simulink model "switch_sample"  (R2021a)
settings: Solver=VariableStepAuto  StartTime=0.0  StopTime=0.5  RelTol=1e-3
settings Model: Creator=Mrittik  LastModifiedBy=Mrittik

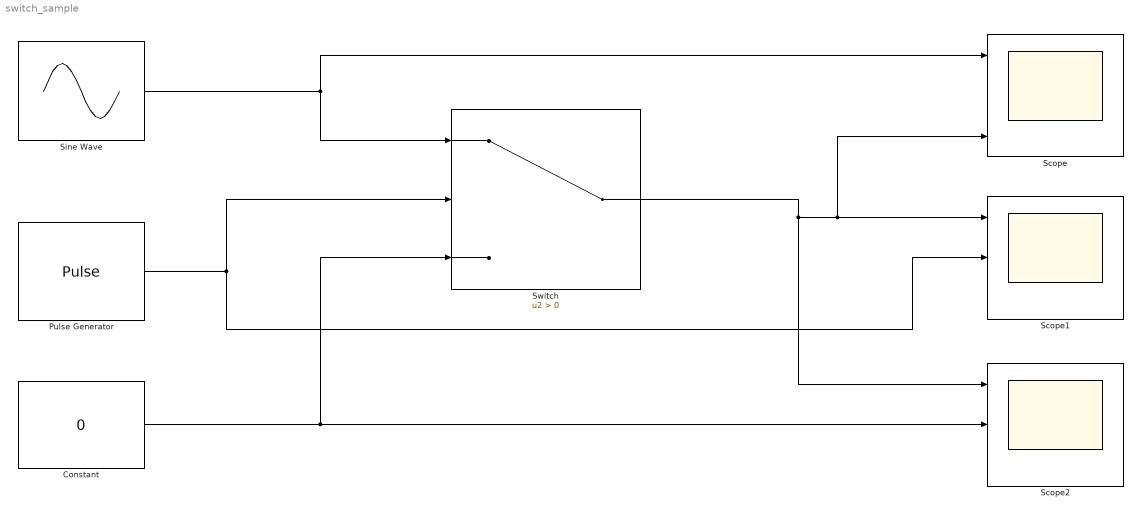
== system switch_sample ==
  Constant : Constant  Value=0  VectorParams1D=off
  Pulse Generator : DiscretePulseGenerator  PulseType=Time based  Period=0.01  PulseWidth=50
  Scope : Scope  NumInputPorts=3
  Scope1 : Scope  NumInputPorts=3
  Scope2 : Scope  NumInputPorts=3
  Sine Wave : Sin  Frequency=100  SampleTime=0
  Switch : Switch  Criteria=u2 > Threshold
  wires:
  Pulse Generator/1 -> Scope1/2, Switch/2
  Constant/1 -> Scope2/2, Switch/3
  Switch/1 -> Scope2/1, Scope1/1, Scope/3
  Sine Wave/1 -> Switch/1, Scope/1
